simulink model "parallel_carrierbased"  (R2016a)
settings: Solver=VariableStepAuto  StartTime=0.0  StopTime=5  RelTol=1e-3
libraries: powerlib x64, powerlib_meascontrol x14, simulink x12
settings Model: Creator=hakan  LastModifiedBy=hakan
settings DataIOCC: LimitDataPoints=on
settings DebuggingCC: AllowSymbolicDim=off
settings ModelReferenceCC: PropagateSignalLabelsOutOfModel=off
settings GRTTargetCC: GeneratePreprocessorConditionals=Use local settings

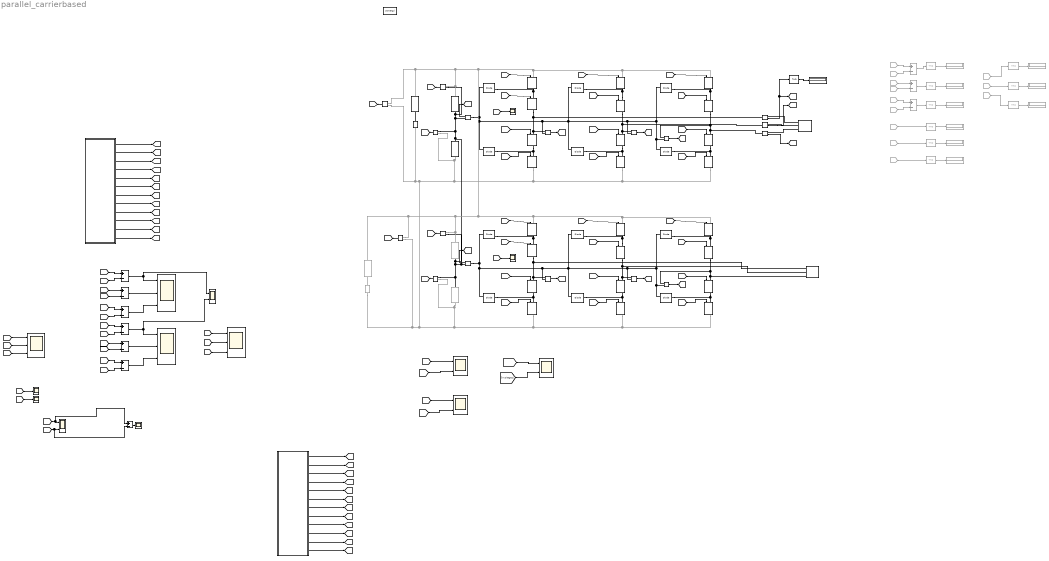
== system parallel_carrierbased ==
  Add{,1..3,7..9} (7 alike) : Sum  Inputs=+-
  Add4 : Sum  Commented=on  Inputs=+-
  Add5 : Sum  Commented=on  Inputs=+-
  Add6 : Sum  Commented=on  Inputs=+-
  Current Measurement{,1..3,5} (5 alike) : powerlib/Measurements/Current Measurement  PhasorSimulation=off  OutputType=Complex  PSBequivalent=0
  DC Voltage Source : powerlib/Electrical Sources/DC Voltage Source  Amplitude=540  Measurements=None
  DC Voltage Source1 : powerlib/Electrical Sources/DC Voltage Source  Commented=on  Amplitude=540  Measurements=None
  Diode{,1..11} (12 alike) : powerlib/Power Electronics/Diode  Ron=0.001  Lon=0  Vf=0.8  IC=0  UseSnubber=off  Rs=500  Cs=250e-9  Measurements=on
  Display : Display
  Display{1..9} (9 alike) : Display  Commented=on
  From26 : From  Commented=on  GotoTag=Ia
  From27 : From  Commented=on  GotoTag=Ib
  From28 : From  Commented=on  GotoTag=Ic
  From36 : From  Commented=on  GotoTag=Van
  From39 : From  Commented=on  GotoTag=Vbn
  From40 : From  Commented=on  GotoTag=Vbn
  From41 : From  Commented=on  GotoTag=Vcn
  From42 : From  Commented=on  GotoTag=Vcn
  From43 : From  Commented=on  GotoTag=Van
  From44 : From  Commented=on  GotoTag=Van
  From45 : From  Commented=on  GotoTag=Vbn
  From46 : From  Commented=on  GotoTag=Vcn
  IGBT/Diode{,1..23} (24 alike) : powerlib/Power Electronics/IGBT//Diode  Ron=1e-3  Rs=1e5  Cs=inf  Measurements=on
  Scope : Scope
  Series RLC Branch : powerlib/Elements/Series RLC Branch  LConnTagsString=__new0  RConnTagsString=__new0  BranchType=C  Resistance=1  Inductance=1e-3  SetiL0=off  InitialCurrent=0  Capacitance=100e-6  Setx0=off  InitialVoltage=200  Measurements=None
  Series RLC Branch1 : powerlib/Elements/Series RLC Branch  LConnTagsString=__new0  RConnTagsString=__new0  BranchType=C  Resistance=1  Inductance=1e-3  SetiL0=off  InitialCurrent=0  Capacitance=100e-6  Setx0=off  InitialVoltage=200  Measurements=None
  Series RLC Branch2 : powerlib/Elements/Series RLC Branch  Commented=on  LConnTagsString=__new0  RConnTagsString=__new0  BranchType=C  Resistance=1  Inductance=1e-3  SetiL0=off  InitialCurrent=0  Capacitance=1000e-6  Setx0=off  InitialVoltage=200  Measurements=None
  Series RLC Branch3 : powerlib/Elements/Series RLC Branch  Commented=on  LConnTagsString=__new0  RConnTagsString=__new0  BranchType=C  Resistance=1  Inductance=1e-3  SetiL0=off  InitialCurrent=0  Capacitance=1000e-6  Setx0=off  InitialVoltage=200  Measurements=None
  Series RLC Branch4 : powerlib/Elements/Series RLC Branch  LConnTagsString=__new0  RConnTagsString=__new0  BranchType=R  Resistance=1  Inductance=1e-3  SetiL0=off  InitialCurrent=0  Capacitance=1000e-6  Setx0=off  InitialVoltage=0  Measurements=None
  Series RLC Branch5 : powerlib/Elements/Series RLC Branch  Commented=on  LConnTagsString=__new0  RConnTagsString=__new0  BranchType=R  Resistance=1  Inductance=1e-3  SetiL0=off  InitialCurrent=0  Capacitance=1000e-6  Setx0=off  InitialVoltage=0  Measurements=None
  Subsystem : Subsystem
  Subsystem1 : Subsystem
  THD : powerlib_meascontrol/Measurements/THD  Freq=50  Ts=0
  THD{1..9} (9 alike) : powerlib_meascontrol/Measurements/THD  Commented=on  Freq=50  Ts=0
  Three-Phase Series RLC Load : powerlib/Elements/Three-Phase Series RLC Load  LConnTagsString=A|B|C  Configuration=Y (floating)  NominalVoltage=1000  Vabc=[1e3 1e3 1e3]  Vabcp=[1e3 1e3 1e3]  NominalFrequency=50  UnbalancedPower=off  ActivePower=8000/2  InductivePower=3870/2  CapacitivePower=0  Pabc=[10e3 9e3 11e3]  QLabc=[100 90 110]  QCabc=[100 90 110]  Pabcp=[10e3 9e3 11e3]  QLabcp=[100 90 110]  QCabcp=[100 90 110]  Measurements=None  LoadType=constant Z
  Three-Phase Series RLC Load1 : powerlib/Elements/Three-Phase Series RLC Load  LConnTagsString=A|B|C  Configuration=Y (floating)  NominalVoltage=1000  Vabc=[1e3 1e3 1e3]  Vabcp=[1e3 1e3 1e3]  NominalFrequency=50  UnbalancedPower=off  ActivePower=8000/2  InductivePower=3870/2  CapacitivePower=0  Pabc=[10e3 9e3 11e3]  QLabc=[100 90 110]  QCabc=[100 90 110]  Pabcp=[10e3 9e3 11e3]  QLabcp=[100 90 110]  QCabcp=[100 90 110]  Measurements=None  LoadType=constant Z
  Vab1 and Vab2 : Scope  NumInputPorts=2
  Voltage Measurement{,1..11} (12 alike) : powerlib/Measurements/Voltage Measurement  PhasorSimulation=off  OutputType=Complex  PSBequivalent=0
  capacitor voltages{,1..3} (4 alike) : Scope  NumInputPorts=2
  line to line : Scope  NumInputPorts=3
  line to line2 : Scope  NumInputPorts=3
  line to neural : Scope  NumInputPorts=3
  neutral current{,1..3} (4 alike) : Scope
  phase currents : Scope  NumInputPorts=3
  powergui : powerlib/powergui  Priority=1  SimulationMode=Continuous  SolverType=Tustin/Backward Euler (TBE)  SampleTime=50e-6  frequency=60  SPID=off  DisableSnubberDevices=off  DisableRonSwitches=off  DisableVfSwitches=off  SwTol=0  DisplayEquations=off  Interpol=off  ExternalGateDelay=off  methode=off  Ts=10  FunctionMessages=off  echomessages=off  HookPort=off  EnableUseOfTLC=off  x0status=blocks  frequencyindice=0  Pbase=100e6  ErrMax=1e-4  Iterations=50  UnitsV=kV  UnitsW=MW  buscounter=0  RestoreLinks=warning  ResistiveCurrentMeasurement=off  Frange=[0:2:500]  Ylog=off  Xlog=on  ShowGrid=off  save=off  variable=ZData  structure=Cap_V_One  ZoomFFT=off  StartTime=3  cycles=50  DisplayStyle=2  fundamental=50  FreqAxis=off  MaxFrequency=2000  frequencyindicesteady=1  RmsSteady=1  display=off
  wires:
  Subsystem/1("Sa1 ") -> [Sa1]
  Subsystem/2("Sa2 ") -> [Sa2]
  Subsystem/3(Sa1Prime) -> [Sa1P]
  Subsystem/4("Sa2Prime ") -> [Sa2P]
  [Sa1] -> IGBT/Diode/1
  [Sa2] -> IGBT/Diode1/1
  [Sa1P] -> IGBT/Diode2/1
  [Sa2P] -> IGBT/Diode3/1
  [Sb1] -> IGBT/Diode4/1
  [Sb2] -> IGBT/Diode5/1
  [Sb1P] -> IGBT/Diode6/1
  [Sb2P] -> IGBT/Diode7/1
  [Sc1] -> IGBT/Diode8/1
  [Sc2] -> IGBT/Diode9/1
  [Sc1P] -> IGBT/Diode10/1
  [Sc2P] -> IGBT/Diode11/1
  Voltage Measurement/1 -> [Van]
  Subsystem/5(Sb1) -> [Sb1]
  Subsystem/6(Sb2) -> [Sb2]
  Subsystem/7("Sb1P ") -> [Sb1P]
  Subsystem/8(Sb2P) -> [Sb2P]
  Subsystem/9("Sc1 ") -> [Sc1]
  Subsystem/10(Sc2) -> [Sc2]
  Subsystem/11(Sc1P) -> [Sc1P]
  Subsystem/12("Sc2P ") -> [Sc2P]
  Voltage Measurement1/1 -> [Vbn]
  Voltage Measurement2/1 -> [Vcn]
  [Van] -> Add/1
  [Vbn] -> Add/2
  Add/1 -> Vab1 and Vab2/2, line to line/1  "Vab"
  [Vbn] -> Add1/1
  [Vcn] -> Add1/2
  Add1/1 -> line to line/2  "Vbc"
  [Vcn] -> Add2/1
  [Van] -> Add2/2
  Add2/1 -> line to line/3  "Vca"
  [Van] -> line to neural/1
  [Vbn] -> line to neural/2
  [Vcn] -> line to neural/3
  Voltage Measurement3/1 -> [upperc]
  Voltage Measurement4/1 -> [lowerc]
  Current Measurement/1 -> [Ineutral]
  [Ineutral] -> neutral current/1
  [Ineutral] -> neutral current1/1
  Current Measurement1/1 -> THD/1, [Ia]
  Current Measurement2/1 -> [Ib]
  Current Measurement3/1 -> [Ic]
  [Ib] -> phase currents/2
  [Ia] -> phase currents/1
  [Ic] -> phase currents/3
  [lowerc] -> Add3/2, capacitor voltages/2  "lowerc"
  Add3/1 -> Scope/1
  [upperc] -> Add3/1, capacitor voltages/1  "upperc"
  THD/1 -> Display/1
  THD1/1 -> Display1/1
  THD2/1 -> Display2/1
  THD3/1 -> Display3/1
  From36/1 -> Add4/1
  From39/1 -> Add4/2
  From40/1 -> Add5/1
  From41/1 -> Add5/2
  From42/1 -> Add6/1
  From43/1 -> Add6/2
  Add4/1 -> THD1/1
  Add5/1 -> THD2/1
  Add6/1 -> THD3/1
  THD5/1 -> Display5/1
  THD6/1 -> Display6/1
  From44/1 -> THD4/1
  From45/1 -> THD5/1
  From46/1 -> THD6/1
  THD4/1 -> Display4/1
  THD7/1 -> Display7/1
  THD8/1 -> Display8/1
  THD9/1 -> Display9/1
  From27/1 -> THD8/1
  From26/1 -> THD7/1
  From28/1 -> THD9/1
  [Sa12] -> IGBT/Diode12/1
  [Sa22] -> IGBT/Diode13/1
  [Sa1P2] -> IGBT/Diode16/1
  [Sa2P2] -> IGBT/Diode17/1
  [Sb12] -> IGBT/Diode18/1
  [Sb22] -> IGBT/Diode19/1
  [Sb1P2] -> IGBT/Diode20/1
  [Sb2P2] -> IGBT/Diode21/1
  [Sc12] -> IGBT/Diode22/1
  [Sc22] -> IGBT/Diode23/1
  [Sc1P2] -> IGBT/Diode14/1
  [Sc2P2] -> IGBT/Diode15/1
  Voltage Measurement5/1 -> [Van2]
  Voltage Measurement6/1 -> [Vbn2]
  Voltage Measurement7/1 -> [Vcn2]
  Voltage Measurement8/1 -> [upperc2]
  Voltage Measurement9/1 -> [lowerc2]
  Current Measurement5/1 -> [Ineutral2]
  [Ineutral] -> neutral current2/1
  [upperc] -> capacitor voltages1/1
  [lowerc] -> capacitor voltages2/1
  [upperc2] -> capacitor voltages1/2
  [lowerc2] -> capacitor voltages2/2
  Subsystem1/1("Sa1 ") -> [Sa12]
  Subsystem1/2("Sa2 ") -> [Sa22]
  Subsystem1/3(Sa1Prime) -> [Sa1P2]
  Subsystem1/4("Sa2Prime ") -> [Sa2P2]
  Subsystem1/5(Sb1) -> [Sb12]
  Subsystem1/6(Sb2) -> [Sb22]
  Subsystem1/7("Sb1P ") -> [Sb1P2]
  Subsystem1/8(Sb2P) -> [Sb2P2]
  Subsystem1/9("Sc1 ") -> [Sc12]
  Subsystem1/10(Sc2) -> [Sc22]
  Subsystem1/11(Sc1P) -> [Sc1P2]
  Subsystem1/12("Sc2P ") -> [Sc2P2]
  Voltage Measurement10/1 -> [involtage2]
  Voltage Measurement11/1 -> [involtage]
  [involtage] -> capacitor voltages3/1
  [involtage2] -> capacitor voltages3/2
  [Van2] -> Add7/1
  [Vbn2] -> Add7/2
  Add7/1 -> Vab1 and Vab2/1, line to line2/1  "Vab"
  [Vbn2] -> Add8/1
  [Vcn2] -> Add8/2
  Add8/1 -> line to line2/2  "Vbc"
  [Vcn2] -> Add9/1
  [Van2] -> Add9/2
  Add9/1 -> line to line2/3  "Vca"
  [Ineutral2] -> neutral current3/1
  connections:
  IGBT/Diode/RConn1 -- Diode/RConn1 -- IGBT/Diode1/LConn1
  IGBT/Diode13/RConn1 -- Three-Phase Series RLC Load1/LConn1 -- IGBT/Diode16/LConn1 -- Voltage Measurement5/LConn1
  IGBT/Diode2/RConn1 -- Diode1/LConn1 -- IGBT/Diode3/LConn1
  IGBT/Diode5/LConn1 -- Diode2/RConn1 -- IGBT/Diode4/RConn1
  IGBT/Diode6/RConn1 -- Diode3/LConn1 -- IGBT/Diode7/LConn1
  IGBT/Diode5/RConn1 -- Current Measurement2/LConn1 -- Voltage Measurement1/LConn1 -- IGBT/Diode6/LConn1
  Diode4/RConn1 -- IGBT/Diode8/RConn1 -- IGBT/Diode9/LConn1
  Diode5/LConn1 -- IGBT/Diode11/LConn1 -- IGBT/Diode10/RConn1
  IGBT/Diode9/RConn1 -- Voltage Measurement2/LConn1 -- Current Measurement3/LConn1 -- IGBT/Diode10/LConn1
  Diode5/RConn1 -- Diode4/LConn1 -- Voltage Measurement1/LConn2 -- Diode3/RConn1 -- Voltage Measurement/LConn2 -- Diode1/RConn1 -- Current Measurement/LConn1 -- Diode/LConn1 -- Diode2/LConn1 -- Voltage Measurement2/LConn2
  Three-Phase Series RLC Load/LConn3 -- Current Measurement3/RConn1
  Three-Phase Series RLC Load/LConn2 -- Current Measurement2/RConn1
  Three-Phase Series RLC Load/LConn1 -- Current Measurement1/RConn1
  IGBT/Diode12/RConn1 -- IGBT/Diode13/LConn1 -- Diode6/RConn1
  IGBT/Diode16/RConn1 -- IGBT/Diode17/LConn1 -- Diode7/LConn1
  IGBT/Diode19/LConn1 -- IGBT/Diode18/RConn1 -- Diode8/RConn1
  IGBT/Diode20/RConn1 -- IGBT/Diode21/LConn1 -- Diode9/LConn1
  Diode10/RConn1 -- IGBT/Diode23/LConn1 -- IGBT/Diode22/RConn1
  Diode11/LConn1 -- IGBT/Diode14/RConn1 -- IGBT/Diode15/LConn1
  Diode11/RConn1 -- Voltage Measurement7/LConn2 -- Diode8/LConn1 -- Diode6/LConn1 -- Current Measurement5/LConn1 -- Diode7/RConn1 -- Voltage Measurement5/LConn2 -- Diode9/RConn1 -- Voltage Measurement6/LConn2 -- Diode10/LConn1
  DC Voltage Source/RConn1 -- Series RLC Branch4/RConn1
  DC Voltage Source1/RConn1 -- Series RLC Branch5/RConn1
  IGBT/Diode23/RConn1 -- Three-Phase Series RLC Load1/LConn3 -- IGBT/Diode14/LConn1 -- Voltage Measurement7/LConn1
  Voltage Measurement6/LConn1 -- Three-Phase Series RLC Load1/LConn2 -- IGBT/Diode19/RConn1 -- IGBT/Diode20/LConn1
  Current Measurement1/LConn1 -- IGBT/Diode1/RConn1 -- Voltage Measurement/LConn1 -- IGBT/Diode2/LConn1
  DC Voltage Source1/LConn1 -- Voltage Measurement9/LConn2 -- Series RLC Branch3/RConn1 -- IGBT/Diode17/RConn1 -- IGBT/Diode21/RConn1 -- IGBT/Diode15/RConn1 -- IGBT/Diode11/RConn1 -- IGBT/Diode7/RConn1 -- IGBT/Diode3/RConn1 -- Series RLC Branch1/RConn1 -- Voltage Measurement4/LConn2 -- Voltage Measurement11/LConn2 -- DC Voltage Source/LConn1 -- Voltage Measurement10/LConn2
  Voltage Measurement9/LConn1 -- Current Measurement5/RConn1 -- Series RLC Branch/RConn1 -- Voltage Measurement3/LConn2 -- Current Measurement/RConn1 -- Voltage Measurement4/LConn1 -- Series RLC Branch1/LConn1 -- Voltage Measurement8/LConn2 -- Series RLC Branch2/RConn1 -- Series RLC Branch3/LConn1
  Series RLC Branch5/LConn1 -- IGBT/Diode22/LConn1 -- IGBT/Diode18/LConn1 -- IGBT/Diode12/LConn1 -- Voltage Measurement11/LConn1 -- Series RLC Branch4/LConn1 -- Series RLC Branch/LConn1 -- Voltage Measurement3/LConn1 -- IGBT/Diode8/LConn1 -- IGBT/Diode4/LConn1 -- IGBT/Diode/LConn1 -- Voltage Measurement8/LConn1 -- Series RLC Branch2/LConn1 -- Voltage Measurement10/LConn1

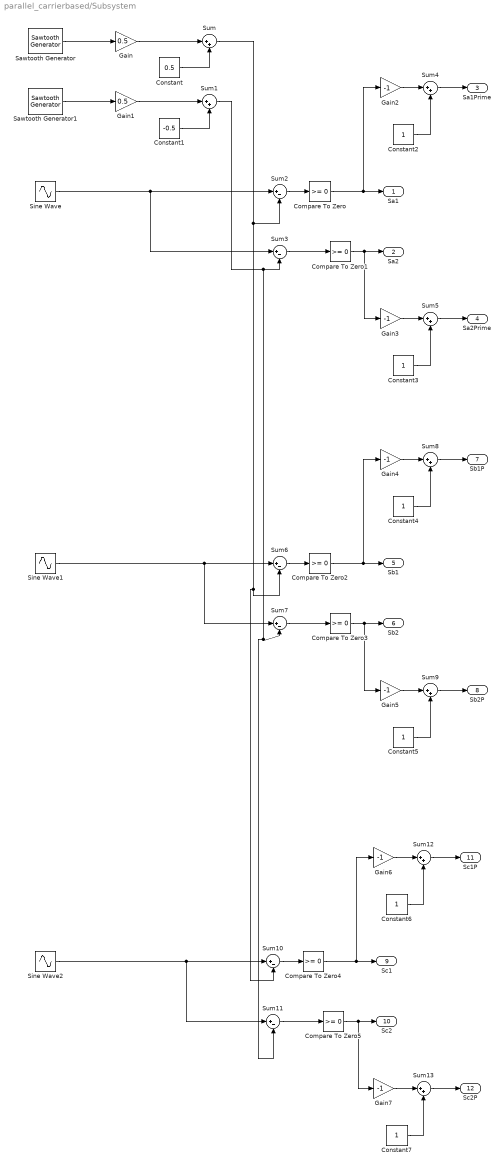
== system parallel_carrierbased/Subsystem ==
  Compare To Zero{,1..5} (6 alike) : simulink/Logic and Bit Operations/Compare To Zero  relop=>=  OutDataTypeStr=boolean
  Constant : Constant  Value=0.5
  Constant1 : Constant  Value=-0.5
  Constant{2..7} (6 alike) : Constant
  Gain : Gain  Gain=0.5
  Gain1 : Gain  Gain=0.5
  Gain{2..7} (6 alike) : Gain  Gain=-1
  Sawtooth Generator : powerlib_meascontrol/Pulse & Signal Generators/Sawtooth Generator  Freq=2050  Phase=180  Ts=0
  Sawtooth Generator1 : powerlib_meascontrol/Pulse & Signal Generators/Sawtooth Generator  Freq=2050  Phase=180  Ts=0
  Sine Wave : Sin  Frequency=100*pi  SampleTime=0
  Sine Wave1 : Sin  Frequency=100*pi  Phase=2*pi/3  SampleTime=0
  Sine Wave2 : Sin  Frequency=100*pi  Phase=4*pi/3  SampleTime=0
  Sum{,1,4..5,8..9,12..13} (8 alike) : Sum  Inputs=|++
  Sum{2..3,6..7,10..11} (6 alike) : Sum  Inputs=|+-
  "Sa1 " : Outport
  "Sa2 " : Outport  Port=2
  Sa1Prime : Outport  Port=3
  "Sa2Prime " : Outport  Port=4
  Sb1 : Outport  Port=5
  Sb2 : Outport  Port=6
  "Sb1P " : Outport  Port=7
  Sb2P : Outport  Port=8
  "Sc1 " : Outport  Port=9
  Sc2 : Outport  Port=10
  Sc1P : Outport  Port=11
  "Sc2P " : Outport  Port=12
  wires:
  Sawtooth Generator/1 -> Gain/1
  Gain/1 -> Sum/1
  Sum/1 -> Sum2/2, Sum10/2, Sum6/2
  Constant/1 -> Sum/2
  Sawtooth Generator1/1 -> Gain1/1
  Gain1/1 -> Sum1/1
  Sum1/1 -> Sum11/2, Sum7/2, Sum3/2
  Constant1/1 -> Sum1/2
  Sine Wave/1 -> Sum3/1, Sum2/1
  Sum2/1 -> Compare To Zero/1
  Compare To Zero/1 -> Gain2/1, "Sa1 "/1
  Sum3/1 -> Compare To Zero1/1
  Compare To Zero1/1 -> Gain3/1, "Sa2 "/1
  Constant2/1 -> Sum4/2
  Gain2/1 -> Sum4/1
  Sum4/1 -> Sa1Prime/1
  Constant3/1 -> Sum5/2
  Gain3/1 -> Sum5/1
  Sum5/1 -> "Sa2Prime "/1
  Sum6/1 -> Compare To Zero2/1
  Compare To Zero2/1 -> Sb1/1, Gain4/1
  Sum7/1 -> Compare To Zero3/1
  Compare To Zero3/1 -> Sb2/1, Gain5/1
  Constant4/1 -> Sum8/2
  Gain4/1 -> Sum8/1
  Sum8/1 -> "Sb1P "/1
  Constant5/1 -> Sum9/2
  Gain5/1 -> Sum9/1
  Sum9/1 -> Sb2P/1
  Sine Wave1/1 -> Sum7/1, Sum6/1
  Sum10/1 -> Compare To Zero4/1
  Compare To Zero4/1 -> Gain6/1, "Sc1 "/1
  Sum11/1 -> Compare To Zero5/1
  Compare To Zero5/1 -> Gain7/1, Sc2/1
  Constant6/1 -> Sum12/2
  Gain6/1 -> Sum12/1
  Sum12/1 -> Sc1P/1
  Constant7/1 -> Sum13/2
  Gain7/1 -> Sum13/1
  Sum13/1 -> "Sc2P "/1
  Sine Wave2/1 -> Sum11/1, Sum10/1

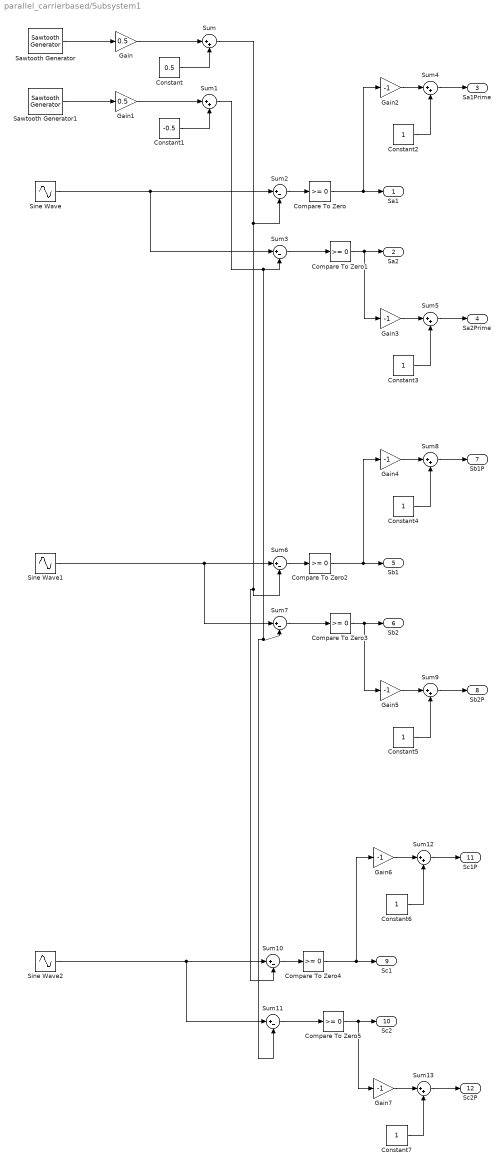
== system parallel_carrierbased/Subsystem1 ==
  Compare To Zero{,1..5} (6 alike) : simulink/Logic and Bit Operations/Compare To Zero  relop=>=  OutDataTypeStr=boolean
  Constant : Constant  Value=0.5
  Constant1 : Constant  Value=-0.5
  Constant{2..7} (6 alike) : Constant
  Gain : Gain  Gain=0.5
  Gain1 : Gain  Gain=0.5
  Gain{2..7} (6 alike) : Gain  Gain=-1
  Sawtooth Generator : powerlib_meascontrol/Pulse & Signal Generators/Sawtooth Generator  Freq=2050  Phase=180  Ts=0
  Sawtooth Generator1 : powerlib_meascontrol/Pulse & Signal Generators/Sawtooth Generator  Freq=2050  Phase=180  Ts=0
  Sine Wave : Sin  Frequency=100*pi  Phase=pi/3  SampleTime=0
  Sine Wave1 : Sin  Frequency=100*pi  Phase=2*pi/3+pi/3  SampleTime=0
  Sine Wave2 : Sin  Frequency=100*pi  Phase=4*pi/3+pi/3  SampleTime=0
  Sum{,1,4..5,8..9,12..13} (8 alike) : Sum  Inputs=|++
  Sum{2..3,6..7,10..11} (6 alike) : Sum  Inputs=|+-
  "Sa1 " : Outport
  "Sa2 " : Outport  Port=2
  Sa1Prime : Outport  Port=3
  "Sa2Prime " : Outport  Port=4
  Sb1 : Outport  Port=5
  Sb2 : Outport  Port=6
  "Sb1P " : Outport  Port=7
  Sb2P : Outport  Port=8
  "Sc1 " : Outport  Port=9
  Sc2 : Outport  Port=10
  Sc1P : Outport  Port=11
  "Sc2P " : Outport  Port=12
  wires:
  Sine Wave2/1 -> Sum10/1, Sum11/1
  Sum13/1 -> "Sc2P "/1
  Gain7/1 -> Sum13/1
  Constant7/1 -> Sum13/2
  Sum12/1 -> Sc1P/1
  Gain6/1 -> Sum12/1
  Constant6/1 -> Sum12/2
  Compare To Zero5/1 -> Sc2/1, Gain7/1
  Sum11/1 -> Compare To Zero5/1
  Compare To Zero4/1 -> "Sc1 "/1, Gain6/1
  Sum10/1 -> Compare To Zero4/1
  Sine Wave1/1 -> Sum6/1, Sum7/1
  Sum9/1 -> Sb2P/1
  Gain5/1 -> Sum9/1
  Constant5/1 -> Sum9/2
  Sum8/1 -> "Sb1P "/1
  Gain4/1 -> Sum8/1
  Constant4/1 -> Sum8/2
  Compare To Zero3/1 -> Gain5/1, Sb2/1
  Sum7/1 -> Compare To Zero3/1
  Compare To Zero2/1 -> Gain4/1, Sb1/1
  Sum6/1 -> Compare To Zero2/1
  Sum5/1 -> "Sa2Prime "/1
  Gain3/1 -> Sum5/1
  Constant3/1 -> Sum5/2
  Sum4/1 -> Sa1Prime/1
  Gain2/1 -> Sum4/1
  Constant2/1 -> Sum4/2
  Compare To Zero1/1 -> "Sa2 "/1, Gain3/1
  Sum3/1 -> Compare To Zero1/1
  Compare To Zero/1 -> "Sa1 "/1, Gain2/1
  Sum2/1 -> Compare To Zero/1
  Sine Wave/1 -> Sum2/1, Sum3/1
  Constant1/1 -> Sum1/2
  Sum1/1 -> Sum3/2, Sum7/2, Sum11/2
  Gain1/1 -> Sum1/1
  Sawtooth Generator1/1 -> Gain1/1
  Constant/1 -> Sum/2
  Sum/1 -> Sum6/2, Sum10/2, Sum2/2
  Gain/1 -> Sum/1
  Sawtooth Generator/1 -> Gain/1
